simulink model "sf_cruise_control_test"  (Simulink 6.0)
settings: Solver=ode45  StartTime=0.0  StopTime=10.0  RelTol=1e-3
PreLoadFcn:
  | Kp = 30; Kd = 30; Ki = 10;
undefined symbols (not defined in the file or in its folder): DiscIntNeverNeededParam, sigbuilder_block
settings Model: CovMetricSettings=dcmtr  Creator=The MathWorks Inc.  LastModifiedBy=batserve  ExtModeAutoUpdateStatusClock=off
settings OptimizationCC: BooleanDataType=off
settings DebuggingCC: CheckExecutionContextPreStartOutputMsg=on  CheckExecutionContextRuntimeOutputMsg=on  SolverPrmCheckMsg=none
settings HardwareCC: TargetUnknown=on

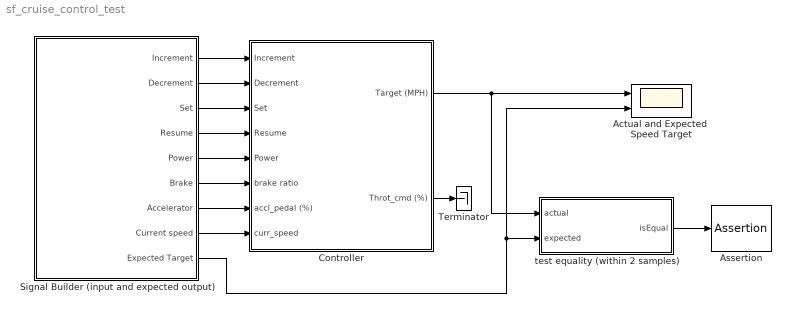
== system sf_cruise_control_test ==
  Actual and Expected  Speed Target : Scope  NumInputPorts=2
      settings: YMin=-1~-1  YMax=35~35
  Assertion : Assertion
  Controller : Subsystem  PropExecContextAcrossSSBoundary=on
  Signal Builder (input and expected output) : Subsystem  Tag=STV Subsys  LoadFcn=sigbuilder_block('load',[38.4 183.2 391.2 268.8 ]);  StartFcn=sigbuilder_block('start');  StopFcn=sigbuilder_block('stop');  ClipboardFcn=sigbuilder_block('clipboard');  PropExecContextAcrossSSBoundary=on
      mask init:
      | tuvar = sigbuilder_block('maskInit');
      settings: CopyFcn=sigbuilder_block('copy');  DeleteFcn=sigbuilder_block('delete');  ModelCloseFcn=sigbuilder_block('modelClose');  PreSaveFcn=sigbuilder_block('preSave');  NameChangeFcn=sigbuilder_block('namechange');  OpenFcn=sigbuilder_block('open',[92.25 347.25 417 342.75 ]);  CloseFcn=sigbuilder_block('close');
      mask Display: plot(0,0,100,100,[10,10,40,40,10],[80,20,20,80,80],[40,10],[50,50], [40,27,10],[65,72,56],[40,25,25,10],[28,28,43,43]);
  Terminator : Terminator
  test equality (within 2 samples) : Subsystem  PropExecContextAcrossSSBoundary=on
  wires:
  Signal Builder (input and expected output)/1(Increment) -> Controller/1(Increment)
  Signal Builder (input and expected output)/2(Decrement) -> Controller/2(Decrement)
  Signal Builder (input and expected output)/3(Set) -> Controller/3(Set)
  Signal Builder (input and expected output)/4(Resume) -> Controller/4(Resume)
  Signal Builder (input and expected output)/5(Power) -> Controller/5(Power)
  Signal Builder (input and expected output)/6(Brake) -> Controller/6(brake ratio)
  Signal Builder (input and expected output)/7(Accelerator) -> Controller/7(accl_pedal (%))
  Signal Builder (input and expected output)/8(Current speed) -> Controller/8(curr_speed)
  Controller/1(Target (MPH)) -> Actual and Expected  Speed Target/1, test equality (within 2 samples)/1(actual)
  Signal Builder (input and expected output)/9(Expected Target) -> test equality (within 2 samples)/2(expected), Actual and Expected  Speed Target/2
  test equality (within 2 samples)/1(isEqual) -> Assertion/1
  Controller/2(Throt_cmd (%)) -> Terminator/1

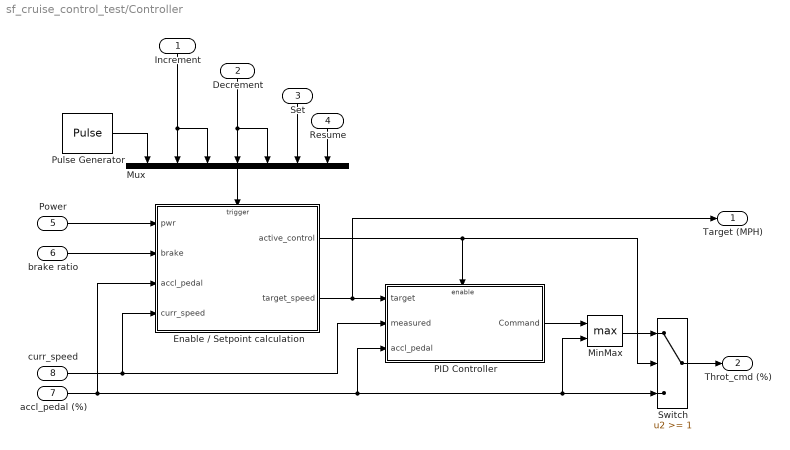
== system sf_cruise_control_test/Controller ==
  Increment : Inport  Orientation=down  Port=1  LatchInput=off
  Decrement : Inport  Orientation=down  Port=2  LatchInput=off
  Set : Inport  Orientation=down  Port=3  LatchInput=off
  Resume : Inport  Orientation=down  Port=4  LatchInput=off
  Power : Inport  Port=5  LatchInput=off
  brake ratio : Inport  Port=6  LatchInput=off
  accl_pedal (%) : Inport  Port=7  LatchInput=off
  curr_speed : Inport  Port=8  LatchInput=off
  Enable / Setpoint calculation : Stateflow chart  TreatAsAtomicUnit=on  PropExecContextAcrossSSBoundary=on
  MinMax : MinMax  Function=max  Inputs=2  ZeroCross=off  SaturateOnIntegerOverflow=on  InputSameDT=on
  Mux : Mux  Orientation=down  Inputs=7
  PID Controller : Subsystem  TreatAsAtomicUnit=on  PropExecContextAcrossSSBoundary=on
  Pulse Generator : DiscretePulseGenerator  SampleTime=.05
  Switch : Switch  Threshold=1  ZeroCross=off  InputSameDT=on
  Target (MPH) : Outport
  Throt_cmd (%) : Outport  Port=2
  wires:
  Mux/1 -> Enable / Setpoint calculation/Trigger
  Enable / Setpoint calculation/2(target_speed) -> PID Controller/1(target), Target (MPH)/1
  curr_speed/1 -> PID Controller/2(measured), Enable / Setpoint calculation/4(curr_speed)
  accl_pedal (%)/1 -> Enable / Setpoint calculation/3(accl_pedal), PID Controller/3(accl_pedal), Switch/3, MinMax/2
  Increment/1 -> Mux/3, Mux/2
  Decrement/1 -> Mux/5, Mux/4
  Set/1 -> Mux/6
  Resume/1 -> Mux/7
  Power/1 -> Enable / Setpoint calculation/1(pwr)
  brake ratio/1 -> Enable / Setpoint calculation/2(brake)
  Switch/1 -> Throt_cmd (%)/1
  Enable / Setpoint calculation/1(active_control) -> Switch/2, PID Controller/Enable
  MinMax/1 -> Switch/1
  PID Controller/1(Command) -> MinMax/1
  Pulse Generator/1 -> Mux/1

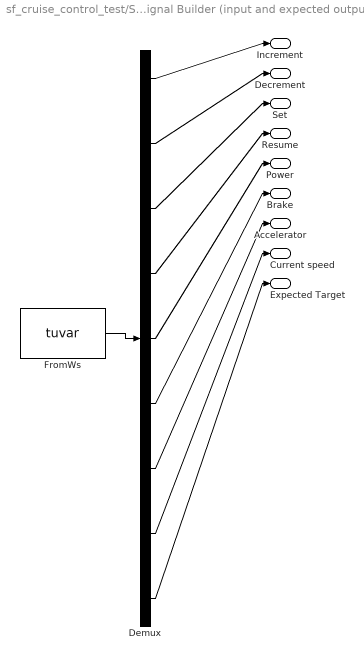
== system sf_cruise_control_test/Signal Builder (input and expected output) ==
  Demux : Demux  Tag=STV Demux  Outputs=9
  FromWs : FromWorkspace  Tag=STV FromWs  VariableName=tuvar  SampleTime=0  OutputAfterFinalValue=Holding final value  SigBuilderData=DataTag0
      SigBuilderData=|
      | channels(1).label = 'Increment'
      | channels(1).allXData = {[0 4 6 10], [0 4 4 5.2 5.2 6 6 7 7 7.5 7.5 8 8 8.5 8.5 10], [0 4 5.2 5.2 6 6 7 7 7.5 7.5 8 8 8.5 8.5 10], [0 3 3 9.5 9.5 10], [0 10], [0 10], [0 4 6 10]}
      | channels(1).allYData = {[0 0 0 0], [0 0 0 0 1 1 0 0 1 1 0 0 1 1 0 0], [0 0 0 1 1 0 0 1 1 0 0 1 1 0 0], [0 0 1 1 0 0], [0 0], [0 0], [0 0 0 0]}
      | channels(2).label = 'Decrement'
      | channels(2).allXData = {[0 10], [0 10], [0 10], [0 10], [0 4 5.2 5.2 6 6 7 7 7.5 7.5 8 8 8.5 8.5 10], [0 3 3 9.5 9.5 10], [0 10]}
      | channels(2).allYData = {[0 0], [0 0], [0 0], [0 0], [0 0 0 1 1 0 0 1 1 0 0 1 1 0 0], [0 0 1 1 0 0], [0 0]}
      | channels(3).label = 'Set'
      | channels(3).allXData = {[0 3 3 10], [0 3 3 10], [0 3 3 10], [0 2 2 10], [0 3 3 10], [0 2 2 10], [0 0.98 0.98 4.02 4.02 10]}
      | channels(3).allYData = {[0 0 1 1], [0 0 1 1], [0 0 1 1], [0 0 1 1], [0 0 1 1], [0 0 1 1], [0 0 1 1 0 0]}
      | channels(4).label = 'Resume'
      | channels(4).allXData = {[0 10], [0 9 9 10], [0 10], [0 10], [0 10], [0 10], [0 7 7 10]}
      | channels(4).allYData = {[0 0], [0 0 1 1], [0 0], [0 0], [0 0], [0 0], [0 0 1 1]}
      | channels(5).label = 'Power'
      | channels(5).allXData = {[0 1 1 10], [0 1 1 10], [0 1 1 10], [0 1 1 10], [0 1 1 10], [0 1 1 10], [0 0.52 0.52 10]}
      | channels(5).allYData = {[0.1 0.1 1 1], [0.1 0.1 1 1], [0.1 0.1 1 1], [0.1 0.1 1 1], [0.1 0.1 1 1], [0.1 0.1 1 1], [0.1 0.1 1 1]}
      | channels(6).label = 'Brake'
      | channels(6).allXData = {[0 10], [0 10], [0 10], [0 10], [0 10], [0 10], [0 3 3 3.5 3.5 5 5 5.5 5.5 10]}
      | channels(6).allYData = {[0 0], [0 0], [0 0], [0 0], [0 0], [0 0], [0 0 0.7 0.7 0 0 0.7 0.7 0 0]}
      | channels(7).label = 'Accelerator'
      | channels(7).allXData = {[0 10], [0 10], [0 10], [0 10], [0 10], [0 10], [0 10]}
      | channels(7).allYData = {[0 0], [0 0], [0 0], [0 0], [0 0], [0 0], [0 0]}
      | channels(8).label = 'Current speed'
      | channels(8).allXData = {[0 10], [0 10], [0 10], [0 10], [0 10], [0 10], [0 10]}
      | channels(8).allYData = {[30 30], [30 30], [30 30], [30 30], [30 30], [30 30], [30 30]}
      | channels(9).label = 'Expected Target'
      | channels(9).allXData = {[0 3 3 10], [0 3 3 5.2 5.2 7 7 8 8 9 9 10], [0 3 3 5.2 5.2 7 7 8 8 9 10], [0 2 2 3 3 4 4 5 5 6 6 7 7 8 8 9 9 10], [0 3 3 5.2 5.2 7 7 8 8 9 10], [0 2 2 3 3 4 4 5 5 6 6 7 7 8 8 9 9 10], [0 1 1 3 3 4 4 5 5 7 7 10]}
      | channels(9).allYData = {[0 0 30 30], [0 0 30 30 31 31 32 32 33 33 30 30], [0 0 30 30 31 31 32 32 33 33 33], [0 0 30 30 31 31 32 32 33 33 34 34 35 35 36 36 37 37], [0 0 30 30 29 29 28 28 27 27 27], [0 0 30 30 29 29 28 28 27 27 26 26 25 25 24 24 23 23], [0 0 30 30 0 0 30 30 0 0 30 30]}
      | common.afterFinalStr = 'Hold final value'
      | common.sampleTime = 0
      | dataSet(1).timeRange = [0 10]
      | dataSet(1).name = 'Reqs. 1,2,8 (power and set)'
      | dataSet(2).timeRange = [0 10]
      | dataSet(2).name = 'Req. 3 (resume)'
      | dataSet(3).timeRange = [0 10]
      | dataSet(3).name = 'Req. 4 (press inc)'
      | dataSet(4).timeRange = [0 10]
      | dataSet(4).name = 'Req. 5 (hold inc)'
      | dataSet(5).timeRange = [0 10]
      | dataSet(5).name = 'Req. 6 (press dec)'
      | dataSet(6).timeRange = [0 10]
      | dataSet(6).name = 'Req. 7 (hold dec)'
      | dataSet(7).timeRange = [0 10]
      | dataSet(7).name = 'Reqs.9,10 (brake, resume)'
  Increment : Outport  Tag=STV Outport
  Decrement : Outport  Tag=STV Outport  Port=2
  Set : Outport  Tag=STV Outport  Port=3
  Resume : Outport  Tag=STV Outport  Port=4
  Power : Outport  Tag=STV Outport  Port=5
  Brake : Outport  Tag=STV Outport  Port=6
  Accelerator : Outport  Tag=STV Outport  Port=7
  Current speed : Outport  Tag=STV Outport  Port=8
  Expected Target : Outport  Tag=STV Outport  Port=9
  wires:
  Demux/9 -> Expected Target/1
  Demux/8 -> Current speed/1
  Demux/7 -> Accelerator/1
  Demux/6 -> Brake/1
  Demux/5 -> Power/1
  Demux/4 -> Resume/1
  Demux/3 -> Set/1
  Demux/2 -> Decrement/1
  Demux/1 -> Increment/1
  FromWs/1 -> Demux/1

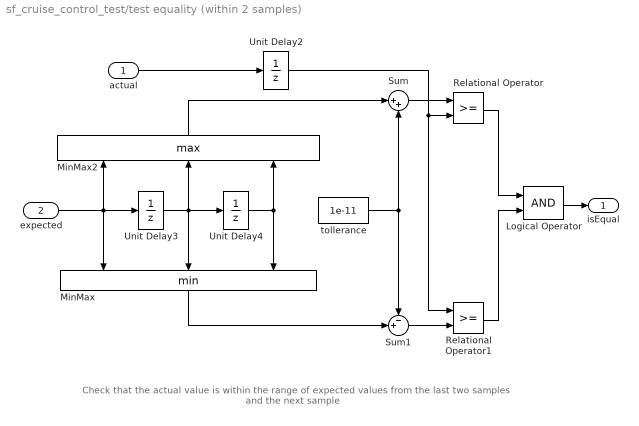
== system sf_cruise_control_test/test equality (within 2 samples) ==
  note: Check that the actual value is within the range of expected
      | values from the last two samples and the next sample
  actual : Inport  Port=1  LatchInput=off
  expected : Inport  Port=2  LatchInput=off
  Logical Operator : Logic
  MinMax : MinMax  Orientation=down  Inputs=3  ZeroCross=off  SaturateOnIntegerOverflow=on  InputSameDT=on
  MinMax2 : MinMax  Orientation=up  Function=max  Inputs=3  ZeroCross=off  SaturateOnIntegerOverflow=on  InputSameDT=on
  Relational Operator : RelationalOperator  ZeroCross=off  InputSameDT=on
  Relational Operator1 : RelationalOperator  ZeroCross=off  InputSameDT=on
  Sum : Sum  Inputs=|++  SaturateOnIntegerOverflow=on  InputSameDT=on
  Sum1 : Sum  Inputs=-+|  SaturateOnIntegerOverflow=on  InputSameDT=on
  Unit Delay2 : UnitDelay  SampleTime=0.1
  Unit Delay3 : UnitDelay  SampleTime=0.1
  Unit Delay4 : UnitDelay  SampleTime=0.1
  tollerance : Constant  Value=1e-11
  isEqual : Outport
  wires:
  Logical Operator/1 -> isEqual/1
  actual/1 -> Unit Delay2/1
  Relational Operator1/1 -> Logical Operator/2
  Relational Operator/1 -> Logical Operator/1
  expected/1 -> Unit Delay3/1, MinMax/1, MinMax2/1
  Unit Delay3/1 -> Unit Delay4/1, MinMax/2, MinMax2/2
  Unit Delay2/1 -> Relational Operator1/1, Relational Operator/2
  Unit Delay4/1 -> MinMax2/3, MinMax/3
  MinMax2/1 -> Sum/1
  Sum/1 -> Relational Operator/1
  Sum1/1 -> Relational Operator1/2
  MinMax/1 -> Sum1/2
  tollerance/1 -> Sum1/1, Sum/2

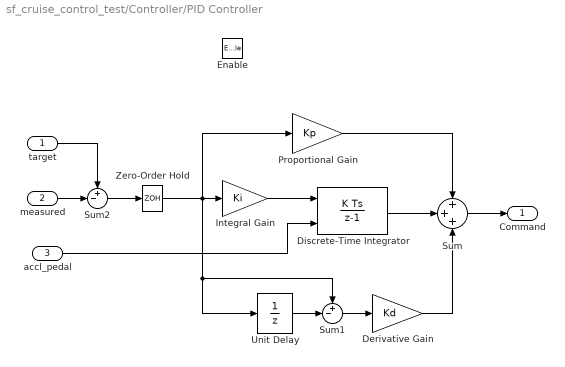
== system sf_cruise_control_test/Controller/PID Controller ==
  target : Inport  Port=1  LatchInput=off
  measured : Inport  Port=2  LatchInput=off
  accl_pedal : Inport  Port=3  LatchInput=off
  Enable : EnablePort  StatesWhenEnabling=reset  ZeroCross=off
  Derivative Gain : Gain  Gain=Kd  SaturateOnIntegerOverflow=on
  Discrete-Time Integrator : DiscreteIntegrator  InitialConditionSource=external  SampleTime=0.1  UpperSaturationLimit=20  LowerSaturationLimit=-20  ICPrevOutput=DiscIntNeverNeededParam  ICPrevScaledInput=DiscIntNeverNeededParam
  Integral Gain : Gain  Gain=Ki  SaturateOnIntegerOverflow=on
  Proportional Gain : Gain  Gain=Kp  SaturateOnIntegerOverflow=on
  Sum : Sum  Inputs=+++  SaturateOnIntegerOverflow=on  InputSameDT=on
  Sum1 : Sum  Inputs=+-|  SaturateOnIntegerOverflow=on  InputSameDT=on
  Sum2 : Sum  Inputs=+-|  SaturateOnIntegerOverflow=on  InputSameDT=on
  Unit Delay : UnitDelay  SampleTime=0.1
  Zero-Order Hold : ZeroOrderHold  SampleTime=0.1
  Command : Outport
  wires:
  Unit Delay/1 -> Sum1/2
  Sum1/1 -> Derivative Gain/1
  Discrete-Time Integrator/1 -> Sum/2
  Derivative Gain/1 -> Sum/3
  Proportional Gain/1 -> Sum/1
  Sum2/1 -> Zero-Order Hold/1
  Sum/1 -> Command/1
  target/1 -> Sum2/1
  measured/1 -> Sum2/2
  Integral Gain/1 -> Discrete-Time Integrator/1
  accl_pedal/1 -> Discrete-Time Integrator/2
  Zero-Order Hold/1 -> Proportional Gain/1, Unit Delay/1, Sum1/1, Integral Gain/1

== stateflow chart Controller/Enable / Setpoint calculation ==
  state Set_Point_Calculation [parallel]
    state Hold
      Hold -> (junction 13) : Set [pwr]
          | {
          | target_speed = curr_speed;
          | set_speed = curr_speed;
          | }
      Hold -> (junction 14) : Resume [pwr]
      (junction 14) -> (junction 15)
      (junction 14) -> (junction 15) : [set_speed > 0]
          |
          | {target_speed = ...
          | set_speed;}
    state Increment
      en: target_speed++;
      Increment -> Increment : every(10,Update)
          | {target_speed++;}
    state Decrement
      en: target_speed--;
      Decrement -> Decrement : every(10,Update)
          | {target_speed--;}
    (default) -> Hold
    Hold -> Increment : INC_BD
        | [in(active_control)]
    Increment -> Hold : INC_BU
    Decrement -> Hold : DEC_BU
    Hold -> Decrement : DEC_BD
        | [in(active_control)]
  state Enable_logic [parallel]
    state Off
    state on
      state active_control
      state overide
        target_speed = 0;
      state no_target
      no_target -> active_control : Set
      (default) -> no_target
      active_control -> overide : [brake]
      overide -> active_control : Set | Resume
    on -> Off : [!pwr]
    Off -> on : [pwr]
    (default) -> Off
  data: pwr input boolean; brake input boolean; accl_pedal input double; active_control output State; target_speed output double; set_speed local double; curr_speed input double
  events: Update input RISING_EDGE_EVENT; INC_BD input RISING_EDGE_EVENT; INC_BU input FALLING_EDGE_EVENT; DEC_BD input RISING_EDGE_EVENT; DEC_BU input FALLING_EDGE_EVENT; Set input EITHER_EDGE_EVENT; Resume input EITHER_EDGE_EVENT
